simulink model "SIMULINKLQG"  (R2025a)
settings: Solver=ode4  StartTime=0.0  StopTime=700  RelTol=1e-3
undefined symbols (not defined in the file): A, A01, A02, At1, At2, B, DiscIntNeverNeededParam, g, K, Kp, L, Veq, Xeq
settings Model: Creator=LENOVO  LastModifiedBy=LENOVO

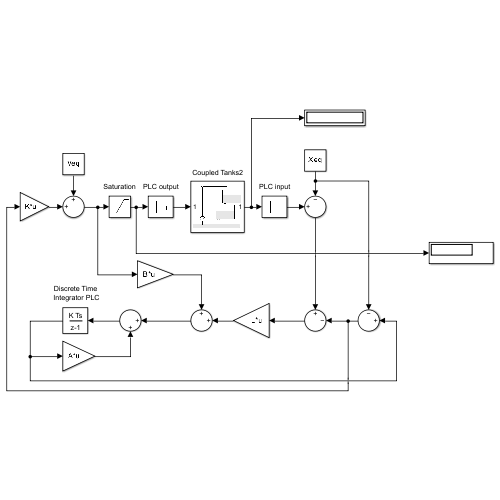
[thumbnail: Simulink's stored preview of the top-level diagram]
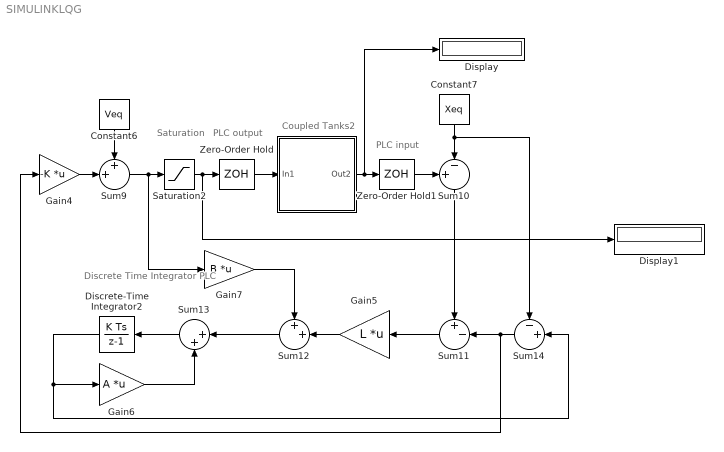
== system SIMULINKLQG ==
  note: PLC input
  note: Coupled Tanks2
  note: Saturation
  note: Discrete Time
      | Integrator PLC
  note: PLC output
  "   " : Subsystem
      mask Display: image('WhatsApp Image 2026-02-13 at 1.35.05 AM.jpeg', [0,0,0,0,95,95]);
  Constant6 : Constant  Value=Veq
  Constant7 : Constant  Value=Xeq
  Discrete-Time Integrator2 : DiscreteIntegrator  SampleTime=0.1  ICPrevOutput=DiscIntNeverNeededParam  ICPrevScaledInput=DiscIntNeverNeededParam
  Display : Display
  Display1 : Display
  Gain4 : Gain  Gain=-K  Multiplication=Matrix(K*u)
  Gain5 : Gain  Gain=L  Multiplication=Matrix(K*u)
  Gain6 : Gain  Gain=A  Multiplication=Matrix(K*u)
  Gain7 : Gain  Gain=B  Multiplication=Matrix(K*u)
  Saturation2 : Saturate  UpperLimit=12  LowerLimit=0
  Sum10 : Sum  Inputs=+-|
  Sum11 : Sum  Inputs=+-|
  Sum12 : Sum  Inputs=++|
  Sum13 : Sum  Inputs=|++
  Sum14 : Sum  Inputs=-+|
  Sum9 : Sum  Inputs=++|
  Zero-Order Hold : ZeroOrderHold  SampleTime=-1
  Zero-Order Hold1 : ZeroOrderHold  SampleTime=-1
  wires:
  Gain7/1 -> Sum12/1
  Constant6/1 -> Sum9/1
  Gain5/1 -> Sum12/2
  Sum13/1 -> Discrete-Time Integrator2/1
  Discrete-Time Integrator2/1 -> Sum14/2, Gain6/1
  Sum9/1 -> Saturation2/1, Gain7/1
  Sum11/1 -> Gain5/1
  Gain4/1 -> Sum9/2
  Sum10/1 -> Sum11/1
  Gain6/1 -> Sum13/2
  Constant7/1 -> Sum10/2, Sum14/1
  Sum12/1 -> Sum13/1
  Sum14/1 -> Sum11/2, Gain4/1
  "   "/1(Out2) -> Display/1, Zero-Order Hold1/1
  Zero-Order Hold/1 -> "   "/1(In1)
  Saturation2/1 -> Display1/1, Zero-Order Hold/1
  Zero-Order Hold1/1 -> Sum10/1

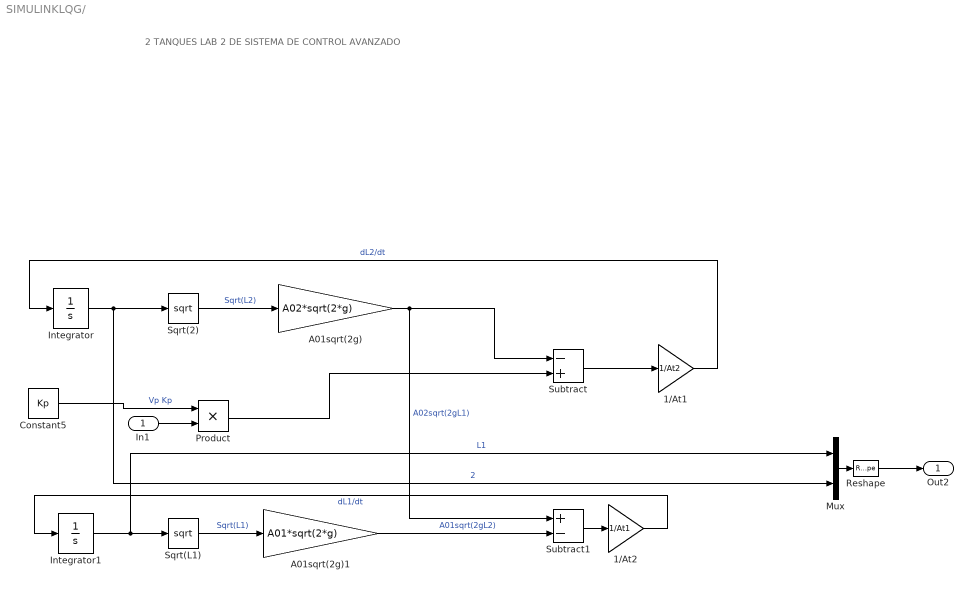
== system SIMULINKLQG/    ==
  note: 2 TANQUES LAB 2 DE SISTEMA DE CONTROL AVANZADO
  In1 : Inport
  1/At1 : Gain  Gain=1/At2
  1/At2 : Gain  Gain=1/At1
  A01sqrt(2g) : Gain  Gain=A02*sqrt(2*g)
  A01sqrt(2g)1 : Gain  Gain=A01*sqrt(2*g)
  Constant5 : Constant  Value=Kp
  Integrator : Integrator
  Integrator1 : Integrator
  Mux : Mux  Inputs=2
  Product : Product
  Reshape : Reshape  OutputDimensionality=Customize  OutputDimensions=[2,1]
  Sqrt(2) : Sqrt
  Sqrt(L1) : Sqrt
  Subtract : Sum  Inputs=-+
  Subtract1 : Sum  Inputs=+-
  Out2 : Outport
  wires:
  Subtract1/1 -> 1/At2/1
  1/At1/1 -> Integrator/1  "dL2/dt"
  1/At2/1 -> Integrator1/1  "dL1/dt"
  Sqrt(2)/1 -> A01sqrt(2g)/1  "Sqrt(L2)"
  Integrator/1 -> Mux/2, Sqrt(2)/1  "2"
  A01sqrt(2g)1/1 -> Subtract1/2  "A01sqrt(2gL2)"
  Integrator1/1 -> Mux/1, Sqrt(L1)/1  "L1"
  A01sqrt(2g)/1 -> Subtract1/1, Subtract/1  "A02sqrt(2gL1)"
  Subtract/1 -> 1/At1/1
  Sqrt(L1)/1 -> A01sqrt(2g)1/1  "Sqrt(L1)"
  Product/1 -> Subtract/2
  Constant5/1 -> Product/1  "Vp Kp"
  In1/1 -> Product/2
  Mux/1 -> Reshape/1
  Reshape/1 -> Out2/1
